simulink model "SMC"  (R2026b)
settings: Solver=ode4  StopTime=8  FixedStep=0.0001
settings Model: Creator=nestorhernandezcastellanos  LastModifiedBy=nestorhernandezcastellanos

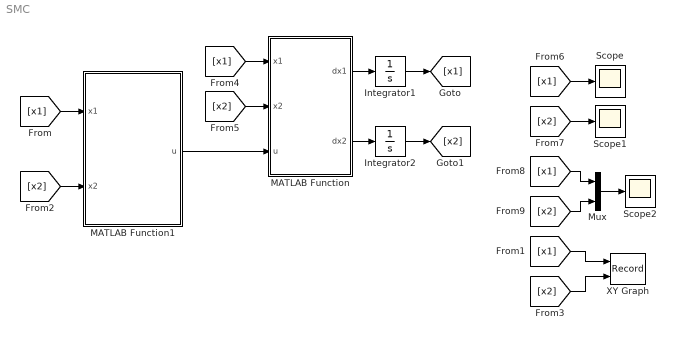
== system SMC ==
  Integrator1 : Integrator  InitialCondition=1
  Integrator2 : Integrator  InitialCondition=-5
  MATLAB Function : MATLAB Function  TreatAsAtomicUnit=on
  MATLAB Function1 : MATLAB Function  TreatAsAtomicUnit=on
  Mux : Mux  Inputs=2
  Scope : Scope
      settings: ActiveDisplayYMinimum=-0.1245779244402196  ActiveDisplayYMaximum=1.12495310271558
  Scope1 : Scope
      settings: ActiveDisplayYMinimum=-1  ActiveDisplayYMaximum=1
  Scope2 : Scope
      settings: ActiveDisplayYMinimum=-5.754762274499031  ActiveDisplayYMaximum=1.7928604704912785  DataLoggingVariableName=ScopeData2
  XY Graph : Record  NumPorts=2.0  FileSettingsInternal="{\"entries\":[{\"content\":{\"excelSettings\":{\"content\":{},\"type\":\"Streamout.ExcelSettings\"},\"parquetSettings\":{\"content\":{},\"type\":\"Streamout.ParquetSettings\"}},\"type\":\"Streamout.FileSettingStorage\",\"uuid\":\"\"}],\"packageUris\":[\"http:\\/\\/schema.mathworks.com\\/mf0\\/streamout_blocks\\/R2020a\"],\"version\":\"1.0\"}"  FrameSettings=[0, 0]  Layout=[1 1]  SignalsInternal="{\"entries\":[{\"content\":{\"signals\":[{\"content\":{\"blockPath\":[],\"dimensions\":[1],\"domain\":\"\",\"lineColor\":\"#a2142f\",\"plots\":[ 1 ],\"port\":1,\"sid\":[\"\"],\"signalID\":1,\"signalName\":\"Integrator1\"},\"type\":\"RecordBlkView.Signal\",\"uuid\":\"\"},{\"content\":{\"blockPath\":[],\"dimensions\":[1],\"domain\":\"\",\"lineColor\":\"#139fff\",\"plots\":[ 1 ],\"port\":2,\"sid\":[\"\"],\"signalID\":2,\"signalName\":\"Integrator2\"},\"type\":\"RecordBlkView.Signal\",\"uuid\":\"\"}]},\"type\":\"RecordBlkView.InputSignals\",\"uuid\":\"\"}],\"packageUris\":[\"http:\\/\\/schema.mathworks.com\\/mf0\\/streamout_blocks\\/R2020a\"],\"version\":\"1.0\"}"  VisualizationBindings="{\"xyplotplugin\":{\"info\":[{\"series\":[{\"bindingParametersList\":[{\"parameter\":\"X-Axis\",\"signalID\":1,\"signalName\":\"Integrator1\"},{\"parameter\":\"Y-Axis\",\"signalID\":2,\"signalName\":\"Integrator2\"}],\"seriesID\":0}],\"subplotID\":1}]}}"  CompatibilityTag=XY
  wires:
  MATLAB Function1/1(u) -> MATLAB Function/3(u)
  MATLAB Function/2(dx2) -> Integrator2/1
  Integrator2/1 -> [x2]
  MATLAB Function/1(dx1) -> Integrator1/1
  Mux/1 -> Scope2/1
  Integrator1/1 -> [x1]
  [x1] -> MATLAB Function1/1(x1)
  [x2] -> MATLAB Function1/2(x2)
  [x1] -> XY Graph/1
  [x2] -> XY Graph/2
  [x1] -> MATLAB Function/1(x1)
  [x2] -> MATLAB Function/2(x2)
  [x1] -> Scope/1
  [x2] -> Scope1/1
  [x1] -> Mux/1
  [x2] -> Mux/2

== matlab function SMC/MATLAB Function1 ==
  data: x1 input; x2 input; u output
function u = controlador(x1, x2)

% Ganancia K>2
K = 2.1;

% Valor arbitrario positivo
C = 1;

sigma = x2 + C*x1;
u = -C*x2 - K*sign(sigma);

== matlab function SMC/MATLAB Function ==
  data: x1 input; x2 input; dx1 output; u input; dx2 output
function [dx1, dx2] = planta(x1, x2, u)

dx1 = x2;
dx2 = sin(x1+x2) + cos(x1*x2) + u;
